simulink model "TPFA_PLL_Mean"  (R2024b)
settings: Solver=VariableStepAuto  StartTime=0.0  StopTime=50e-2  RelTol=1e-3
undefined symbols (not defined in the file or in its folder): DiscIntNeverNeededParam, dspblkCoreblockFVToolHelper, gcbh
libraries: spsMeanLib x1, slpidlib x1, SignalEditorBlockLib x1
settings Model: Creator=byrin  LastModifiedBy=byrin

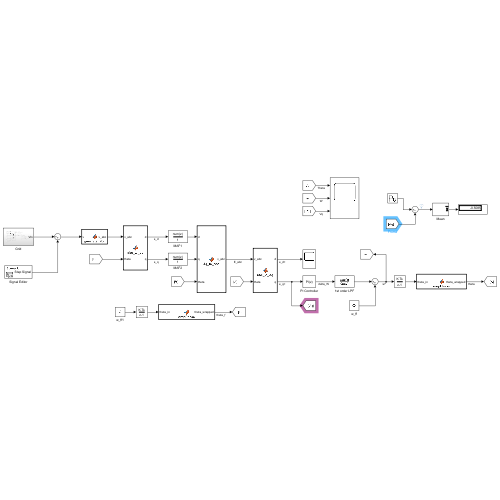
[thumbnail: Simulink's stored preview of the top-level diagram]
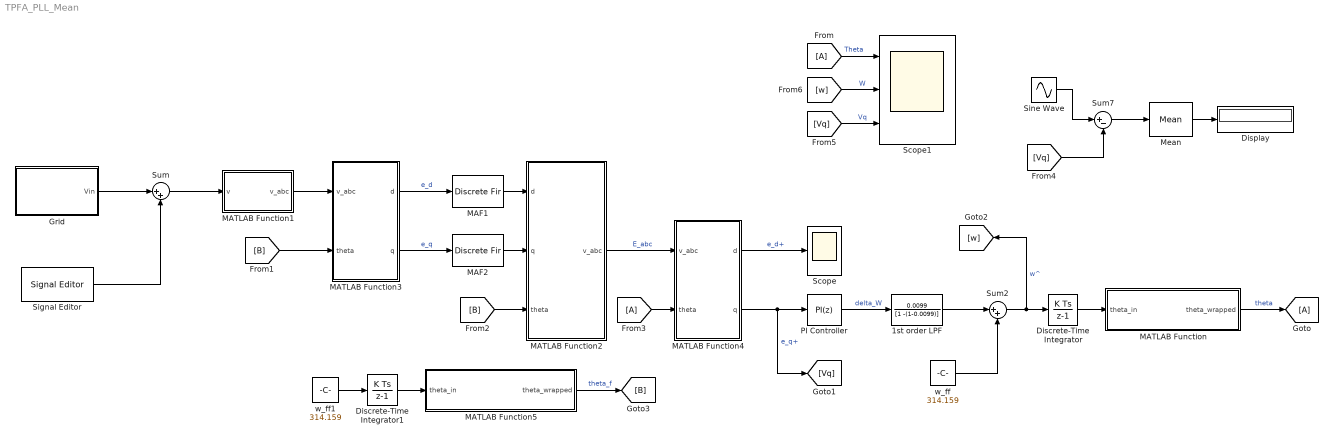
== system TPFA_PLL_Mean ==
  1st order LPF : DiscreteTransferFcn  LoadFcn=dspblkCoreblockFVToolHelper(gcbh,'load');  Numerator=[0.0099]  Denominator=[1 -(1-0.0099)]
      settings: CopyFcn=dspblkCoreblockFVToolHelper(gcbh,'copy');  DeleteFcn=dspblkCoreblockFVToolHelper(gcbh,'close');  ModelCloseFcn=dspblkCoreblockFVToolHelper(gcbh,'close');  PreSaveFcn=dspblkCoreblockFVToolHelper(gcbh,'presave');  PostSaveFcn=dspblkCoreblockFVToolHelper(gcbh,'postsave');  CloseFcn=dspblkCoreblockFVToolHelper(gcbh,'close');
  Discrete-Time Integrator : DiscreteIntegrator  SampleTime=1e-4  ICPrevOutput=DiscIntNeverNeededParam  ICPrevScaledInput=DiscIntNeverNeededParam
  Discrete-Time Integrator1 : DiscreteIntegrator  SampleTime=1e-4  ICPrevOutput=DiscIntNeverNeededParam  ICPrevScaledInput=DiscIntNeverNeededParam
  Display : Display
  From : From
  From3 : From
  Goto : Goto
  Grid : Subsystem
  MAF1 : DiscreteFir  LoadFcn=dspblkCoreblockFVToolHelper(gcbh,'load');  Coefficients=ones(1, 200)/200
      settings: CopyFcn=dspblkCoreblockFVToolHelper(gcbh,'copy');  DeleteFcn=dspblkCoreblockFVToolHelper(gcbh,'close');  ModelCloseFcn=dspblkCoreblockFVToolHelper(gcbh,'close');  PreSaveFcn=dspblkCoreblockFVToolHelper(gcbh,'presave');  PostSaveFcn=dspblkCoreblockFVToolHelper(gcbh,'postsave');  CloseFcn=dspblkCoreblockFVToolHelper(gcbh,'close');
  MAF2 : DiscreteFir  LoadFcn=dspblkCoreblockFVToolHelper(gcbh,'load');  Coefficients=ones(1, 200)/200
      settings: CopyFcn=dspblkCoreblockFVToolHelper(gcbh,'copy');  DeleteFcn=dspblkCoreblockFVToolHelper(gcbh,'close');  ModelCloseFcn=dspblkCoreblockFVToolHelper(gcbh,'close');  PreSaveFcn=dspblkCoreblockFVToolHelper(gcbh,'presave');  PostSaveFcn=dspblkCoreblockFVToolHelper(gcbh,'postsave');  CloseFcn=dspblkCoreblockFVToolHelper(gcbh,'close');
  MATLAB Function : MATLAB Function  TreatAsAtomicUnit=on
  MATLAB Function1 : MATLAB Function  TreatAsAtomicUnit=on
  MATLAB Function2 : MATLAB Function  TreatAsAtomicUnit=on
  MATLAB Function3 : MATLAB Function  TreatAsAtomicUnit=on
  MATLAB Function4 : MATLAB Function  TreatAsAtomicUnit=on
  MATLAB Function5 : MATLAB Function  TreatAsAtomicUnit=on
  Mean : spsMeanLib/Mean  Freq=60  Vinit=0  Ts=0
  PI Controller : slpidlib/PID Controller  Controller=PI  Form=Parallel  TimeDomain=Discrete-time  UseExternalTs=off  SampleTime=1e-4  IntegratorMethod=Forward Euler  FilterMethod=Forward Euler  ControllerParametersSource=internal  P=104  I=4521  UseKiTs=off  D=0  UseExternalDerivativeSource=off  N=100  UseFilter=on  TunerSelectOption=Transfer Function Based (PID Tuner App)  InitialConditionSource=internal  InitialConditionForIntegrator=0  InitialConditionForFilter=0  DifferentiatorICPrevScaledInput=0  ExternalReset=none  TrackingMode=off  Kt=1  LimitOutput=off  SatLimitsSource=internal  UpperSaturationLimit=inf  LowerSaturationLimit=-inf  LinearizeAsGain=on  AntiWindupMode=none  Kb=1  LimitIntegrator=off  UpperIntegratorSaturationLimit=inf  LowerIntegratorSaturationLimit=-inf  POutMin=[]  POutMax=[]  IOutMin=[]  IOutMax=[]  DOutMin=[]  DOutMax=[]  NOutMin=[]  NOutMax=[]  SumOutMin=[]  SumOutMax=[]  SaturationOutMin=[]  SaturationOutMax=[]  PParamMin=[]  PParamMax=[]  IParamMin=[]  IParamMax=[]  DParamMin=[]  DParamMax=[]  NParamMin=[]  NParamMax=[]  KbParamMin=[]  KbParamMax=[]  KtParamMin=[]  KtParamMax=[]  KbOutMin=[]  KbOutMax=[]  KtOutMin=[]  KtOutMax=[]  IntegratorOutMin=[]  IntegratorOutMax=[]  FilterOutMin=[]  FilterOutMax=[]  SumI1OutMin=[]  SumI1OutMax=[]  SumI2OutMin=[]  SumI2OutMax=[]  SumI3OutMin=[]  SumI3OutMax=[]  SumI4OutMin=[]  SumI4OutMax=[]  SumDOutMin=[]  SumDOutMax=[]  DifferentiatorOutMin=[]  DifferentiatorOutMax=[]  FilterDiffOutCoefMin=[]  FilterDiffOutCoefMax=[]  ReciprocalOutMin=[]  ReciprocalOutMax=[]  SumDenOutMin=[]  SumDenOutMax=[]  SumNumOutMin=[]  SumNumOutMax=[]  DivideOutMin=[]  DivideOutMax=[]  UdiffTsProdOutMin=[]  UdiffTsProdOutMax=[]  NTsProdOutMin=[]  NTsProdOutMax=[]  UintegralTsProdOutMin=[]  UintegralTsProdOutMax=[]  UngainTsProdOutMin=[]  UngainTsProdOutMax=[]  ClampingZeroOutDataTypeStr=Inherit: Inherit via back propagation  ClampingZeroOutMin=[]  ClampingZeroOutMax=[]  FilterDenConstantOutDataTypeStr=Inherit: Inherit via back propagation  FilterDenConstantOutMin=[]  FilterDenConstantOutMax=[]  PCopyOutDataTypeStr=Inherit: Inherit via back propagation  PCopyOutMin=[]  PCopyOutMax=[]  NCopyOutDataTypeStr=Inherit: Inherit via back propagation  NCopyOutMin=[]  NCopyOutMax=[]  IntegratorContinuousStateAttributes=''  IntegratorStateMustResolveToSignalObject=off  IntegratorRTWStateStorageClass=Auto  FilterContinuousStateAttributes=''  FilterStateMustResolveToSignalObject=off  FilterRTWStateStorageClass=Auto  ParallelPVariant=InternalParameters  IdealPVariant=Disabled  IVariant=InternalParameters  DVariant=Disabled  IntegratorVariant=Discrete  SatVariant=Disabled  AWVariant=Passthrough  PCopyVariant=Disabled  TRVariant=Disabled  FdbkBlocksVariant=Forward  IdealPFdbkVariant=Disabled  SatFdbkVariant=Disabled  DerivativeFilterVariant=Disabled  NVariant=Disabled  NCopyVariant=Disabled_SignalSpec  FilterICVariant=Disabled  IntegratorICVariant=InternalICs  ExternalResetVariant=Disabled  TRSumVariant=Passthrough  SumFdbkVariant=Disabled  SumVariant=Sum_PI  TsampFilterVariant=InternalTs  TsampNgainVariant=Passthrough  TsampIntegralVariant=Disabled_SignalSpec  ExternalSaturationOutDataTypeStr=Inherit: Same as second input  DerivativeSourceVariant=Disabled  PreIntVariant=InternalPreInt
  Scope : Scope
  Scope1 : Scope  NumInputPorts=3
  Signal Editor : SignalEditorBlockLib/Signal Editor  FileName=Step.mat  ActiveScenario=Scenario  ActiveSignal=Step Signal  IsBus=off  OutputBusObjectStr=Bus: BusObject  SampleTime=1e-4  Interpolate=off  ZeroCross=off  OutputAfterFinalValue=Setting to zero  Unit=inherit  PreserveSignalName=on  ApplySigPropsToAllScenarios=on  ApplySigPropsToAllSignals=off
  Sine Wave : Sin  Frequency=50  SampleTime=1e-4
  Sum : Sum  Inputs=|++
  Sum2 : Sum  Inputs=|++
  Sum7 : Sum  Inputs=|+-
  w_ff : Constant  Value=314.159
  w_ff1 : Constant  Value=314.159
  wires:
  w_ff/1 -> Sum2/2
  MATLAB Function/1(theta_wrapped) -> Goto/1  "theta"
  PI Controller/1 -> 1st order LPF/1  "delta_W"
  Discrete-Time Integrator/1 -> MATLAB Function/1(theta_in)
  Sum2/1 -> [w], Discrete-Time Integrator/1  "w^"
  From/1 -> Scope1/1  "Theta"
  [Vq] -> Scope1/3  "Vq"
  [w] -> Scope1/2  "W"
  1st order LPF/1 -> Sum2/1
  MATLAB Function1/1(v_abc) -> MATLAB Function3/1(v_abc)
  MATLAB Function3/2(q) -> MAF2/1  "e_q"
  MATLAB Function3/1(d) -> MAF1/1  "e_d"
  MAF1/1 -> MATLAB Function2/1(d)
  MAF2/1 -> MATLAB Function2/2(q)
  MATLAB Function2/1(v_abc) -> MATLAB Function4/1(v_abc)  "E_abc"
  From3/1 -> MATLAB Function4/2(theta)
  MATLAB Function4/1(d) -> Scope/1  "e_d+"
  MATLAB Function4/2(q) -> PI Controller/1, [Vq]  "e_q+"
  Discrete-Time Integrator1/1 -> MATLAB Function5/1(theta_in)
  w_ff1/1 -> Discrete-Time Integrator1/1
  MATLAB Function5/1(theta_wrapped) -> [B]  "theta_f"
  [B] -> MATLAB Function3/2(theta)
  [B] -> MATLAB Function2/3(theta)
  Sum/1 -> MATLAB Function1/1(v)
  Grid/1(Vin) -> Sum/1
  Signal Editor/1 -> Sum/2
  Mean/1 -> Display/1
  Sum7/1 -> Mean/1
  Sine Wave/1 -> Sum7/1
  [Vq] -> Sum7/2

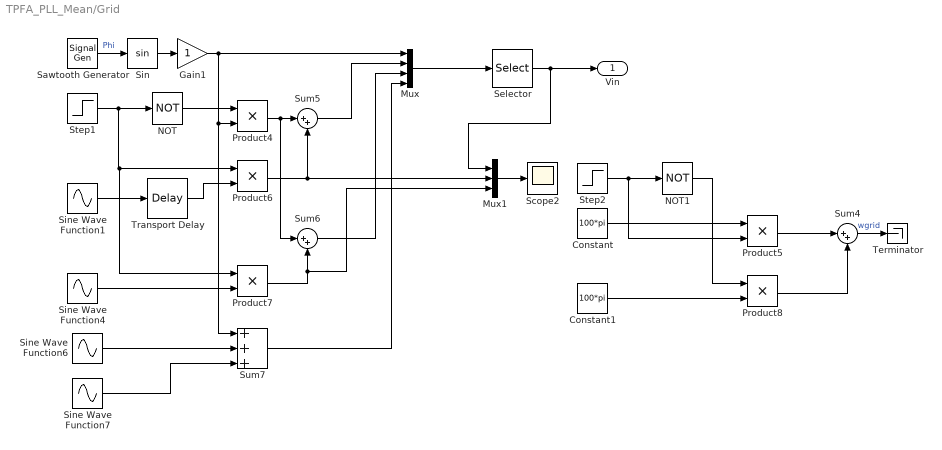
== system TPFA_PLL_Mean/Grid ==
  Constant : Constant  Value=100*pi
  Constant1 : Constant  Value=100*pi
  Gain1 : Gain
  Mux : Mux
  Mux1 : Mux  Inputs=3
  NOT : Logic  Operator=NOT  IconShape=distinctive  AllPortsSameDT=off  OutDataTypeStr=boolean
  NOT1 : Logic  Operator=NOT  IconShape=distinctive  AllPortsSameDT=off  OutDataTypeStr=boolean
  Product{4..8} (5 alike) : Product
  Sawtooth Generator : SignalGenerator  WaveForm=sawtooth  Amplitude=pi  Frequency=314.159  Units=rad/sec
  Scope2 : Scope
  Selector : Selector  InputPortWidth=4  IndexOptions=Index vector (dialog)  Indices=1  OutputSizes=1
  Sin : Trigonometry
  Sine Wave Function1 : Sin  Frequency=314.159  SampleTime=0
  Sine Wave Function4 : Sin  Frequency=314.159  Phase=pi  SampleTime=0
  Sine Wave Function6 : Sin  Amplitude=1*0.1  Frequency=5*100*pi  SampleTime=0
  Sine Wave Function7 : Sin  Amplitude=1*0.05  Frequency=10*100*pi  SampleTime=0
  Step1 : Step  SampleTime=0
  Step2 : Step  Before=1  After=0  SampleTime=0
  Sum4 : Sum  Inputs=|++
  Sum5 : Sum  Inputs=|++
  Sum6 : Sum  Inputs=|++
  Sum7 : Sum  Inputs=+++
  Terminator : Terminator
  Transport Delay : TransportDelay  DelayTime=1000e-3
  Vin : Outport
  wires:
  Product5/1 -> Sum4/1
  NOT/1 -> Product4/1
  Product7/1 -> Mux1/3, Sum6/2
  Sum6/1 -> Mux/3
  Sine Wave Function4/1 -> Product7/2
  Product6/1 -> Mux1/2, Sum5/2
  Sin/1 -> Gain1/1
  Mux1/1 -> Scope2/1
  Sum7/1 -> Mux/4
  Sum4/1 -> Terminator/1  "wgrid"
  NOT1/1 -> Product8/1
  Product4/1 -> Sum6/1, Sum5/1
  Sum5/1 -> Mux/2
  Transport Delay/1 -> Product6/2
  Mux/1 -> Selector/1
  Constant1/1 -> Product8/2
  Step2/1 -> Product5/2, NOT1/1
  Sine Wave Function6/1 -> Sum7/2
  Step1/1 -> Product7/1, Product6/1, NOT/1
  Gain1/1 -> Sum7/1, Product4/2, Mux/1
  Sawtooth Generator/1 -> Sin/1  "Phi"
  Selector/1 -> Vin/1, Mux1/1
  Sine Wave Function7/1 -> Sum7/3
  Constant/1 -> Product5/1
  Product8/1 -> Sum4/2
  Sine Wave Function1/1 -> Transport Delay/1

== matlab function TPFA_PLL_Mean/MATLAB Function ==
  data: theta_in input; theta_wrapped output
function theta_wrapped = wrapPhase(theta_in)
% Wraps phase to [0, 2*pi)
theta_wrapped = mod(theta_in, 2*pi);
end

== matlab function TPFA_PLL_Mean/MATLAB Function2 ==
  data: d input; v_abc output; q input; theta input
function v_abc = dq_to_abc(d, q, theta)

v_alpha = d*cos(theta) - q*sin(theta);
v_beta  = d*sin(theta) + q*cos(theta);

v_abc = zeros(3,1);
v_abc(1) = v_alpha;
v_abc(2) = -0.5*v_alpha + (sqrt(3)/2)*v_beta;
v_abc(3) = -0.5*v_alpha - (sqrt(3)/2)*v_beta;
end

== matlab function TPFA_PLL_Mean/MATLAB Function3 ==
  data: v_abc input; d output; theta input; q output
function [d, q] = abc_to_dq(v_abc, theta)
v_alpha = (2/3)*(v_abc(1) - 0.5*v_abc(2) - 0.5*v_abc(3));
v_beta  = (2/3)*(sqrt(3)/2)*(v_abc(2) - v_abc(3));
d =  v_alpha*cos(theta) + v_beta*sin(theta);
q = -v_alpha*sin(theta) + v_beta*cos(theta);
end

== matlab function TPFA_PLL_Mean/MATLAB Function4 ==
  data: v_abc input; d output; theta input; q output
function [d, q] = abc_to_dq(v_abc, theta)
v_alpha = (2/3)*(v_abc(1) - 0.5*v_abc(2) - 0.5*v_abc(3));
v_beta  = (2/3)*(sqrt(3)/2)*(v_abc(2) - v_abc(3));
d =  v_alpha*cos(theta) + v_beta*sin(theta);
q = -v_alpha*sin(theta) + v_beta*cos(theta);
end

== matlab function TPFA_PLL_Mean/MATLAB Function5 ==
  data: theta_in input; theta_wrapped output
function theta_wrapped = wrapPhase(theta_in)
% Wraps phase to [0, 2*pi)
theta_wrapped = mod(theta_in, 2*pi);
end

== matlab function TPFA_PLL_Mean/MATLAB Function1 ==
  data: v input; v_abc output
function v_abc = generate_abc(v)
v_abc = zeros(3,1);
v_abc(1) = v;                           % v_a
v_abc(2) = v * cos(2*pi/3);            % v_b
v_abc(3) = v * cos(4*pi/3);            % v_c
end
